simulink model "delayedobserver"  (R2016b)
settings: Solver=ode45  StartTime=0.0  StopTime=T  MaxStep=MaxStep  RelTol=RelTol  EnableMultiTasking=on
values from neighbouring files (symbols this model uses):
  J = 50    [ACC2018_1402_workspace.mat]    (also in initialization.m)
  L = [0.77524 0.18123 -0.12123 -0.17406 0.22469]    [ACC2018_1402_workspace.mat]    (also in initialization.m = [0.77524 0.18123 -0.12123 -0.17406 0.22469]')
  Q = [1 0 0 0 1]    [ACC2018_1402_workspace.mat]    (also in initialization.m)
  rule = 1    [ACC2018_1402_workspace.mat]    (also in initialization.m)
  T = 50    [ACC2018_1402_workspace.mat]    (also in initialization.m)
  T1 = 0.2    [ACC2018_1402_workspace.mat]    (also in initialization.m)
  T2 = 3    [ACC2018_1402_workspace.mat]    (also in initialization.m)
  Tdel = 0.15    [ACC2018_1402_workspace.mat]    (also in initialization.m)
  x0 = [1.73848352419 -6.75635383614 5.88569081368 -3.7756991591 0.570662710124 1 2.03963882803 -4.7405743092 3.08158196954 3.7842900628 4.96303185647 0.0125732066995]    [ACC2018_1402_workspace.mat]    (also in initialization.m = [taus0; e0; mu0; tau0])
libraries: simulink x3
settings Model: Creator=pablonanez  LastModifiedBy=Berk
settings DataIOCC: LimitDataPoints=on  SaveFormat=Array  SignalLoggingSaveFormat=ModelDataLogs
settings OptimizationCC: ExpressionDepthLimit=2147483647  LifeSpan=inf
settings DebuggingCC: UnderspecifiedInitializationDetection=Classic  MergeDetectMultiDrivingBlocksExec=none  SolverPrmCheckMsg=warning  FcnCallInpInsideContextMsg=warning  StateNameClashWarn=warning  SFUnexpectedBacktrackingDiag=warning  SFNoUnconditionalDefaultTransitionDiag=warning  SFExecutionAtInitializationDiag=none
settings HardwareCC: ProdBitPerPointer=32  ProdBitPerSizeT=32  ProdBitPerPtrDiffT=32  ProdLargestAtomicFloat=None  ProdIntDivRoundTo=Undefined  ProdEndianess=Unspecified  ProdWordSize=32  ProdHWDeviceType=32-bit Generic
settings ModelReferenceCC: PropagateSignalLabelsOutOfModel=off
settings SFSimCC: SimParseCustomCode=off
settings GRTTargetCC: TargetLangStandard=C89/C90 (ANSI)  GeneratePreprocessorConditionals=Disable all  CombineOutputUpdateFcns=off  GRTInterface=on
settings ConfigComp: CovMetricSettings=dw  CovHtmlReporting=on  CovSaveCumulativeToWorkspaceVar=on  CovSaveSingleToWorkspaceVar=on  CovExternalEMLEnable=off

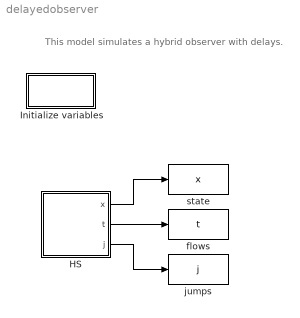
== system delayedobserver ==
  note: This model simulates a hybrid observer with delays.
  HS : Subsystem  LoadFcn=set_param(gcb,'LinkStatus','none')
      settings: CopyFcn=|
      | set_param(gcb,'LinkStatus','none')
      | set_param(gcs, 'MaxStep', 'MaxStep', 'RelTol', 'RelTol')
      mask Display:
      | image(imread('Hcal.jpg'))
      | %plot([5 20 20 5 5],[5 5 20 20 5])
      | %text(8,13,'HyEq_mdl')
      | port_label('output', 1, 'x')
      | port_label('output', 2, 't')
      | port_label('output', 3, 'j')
  Initialize variables : Subsystem  Priority=-10
      settings: OpenFcn=initialization_ex1_4
      mask Display: disp('Double Click\n to Initialize')
  flows : ToWorkspace  VariableName=t  SampleTime=-1
  jumps : ToWorkspace  VariableName=j  SampleTime=-1
  state : ToWorkspace  VariableName=x  SampleTime=-1
  wires:
  HS/1(x) -> state/1
  HS/2(t) -> flows/1
  HS/3(j) -> jumps/1

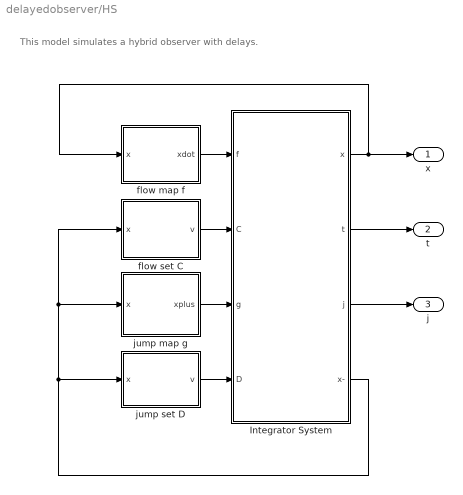
== system delayedobserver/HS ==
  note: This model simulates a hybrid observer with delays.
  Integrator System : Subsystem  Priority=2  mask(Hybrid Integrator){T=T, J=J, x0=x0}
      mask prompts: T "Flow Horizon"; J "Jump Horizon"; x0 "Initial Condition"
      mask help:
      | This block integrates the state of the hybrid system defined by the flow map f (first input), the flow set C (second input), the jump map g (third input) and the jump set D (fourth input).
      | Starting from the initial condition x0 (last mask parameter), the system's state x evolves continuously within the set C, according to f(x,u), but is also subject to jumps within D, according to g(x,u).
      | The block also stops the simulation when the time t is greater than the flow horizon T (first mask parameter), or when the number of jumps j is greater than the jump horizon J (second mask parameter).
      | The outputs of the blocks are respectively x(t), t, j, x(t-).
      mask Help:
      | This block integrates the state of the hybrid system defined by the flow map f (first input), the flow set C (second input), the jump map g (third input) and the jump set D (fourth input).
      | <br>
      | Starting from the initial condition x0 (last mask parameter), the system's state x evolves continuously within the set C, according to f(x,u), but is also subject to jumps within D, according to g(x,u).
      | <br>
      | The block also stops the simulation when the time t is greater than the flow horizon T (first mask parameter), or when the number of jumps j is greater than the jump horizon J (second mask parameter).
      | <br>
      | The outputs of the blocks are respectively x(t), t, j, x(t-).
      | <br>
      | You can right click on the block and "Look under mask" to see what's inside the block.
      | Finally, refer to the manual (HybridSimulator_vXX.pdf) for more detailed information on how this hybrid simulator works.
  flow map f : MATLAB Function  TreatAsAtomicUnit=on
  flow set C : MATLAB Function  TreatAsAtomicUnit=on
  jump map g : MATLAB Function  Priority=2  TreatAsAtomicUnit=on
  jump set D : MATLAB Function  TreatAsAtomicUnit=on
  x : Outport
  t : Outport  Port=2
  j : Outport  Port=3
  wires:
  flow map f/1(xdot) -> Integrator System/1(f)
  Integrator System/4(x-) -> jump set D/1(x), flow set C/1(x), jump map g/1(x)
  Integrator System/1(x) -> flow map f/1(x), x/1
  flow set C/1(v) -> Integrator System/2(C)
  Integrator System/2(t) -> t/1
  Integrator System/3(j) -> j/1
  jump set D/1(v) -> Integrator System/4(D)
  jump map g/1(xplus) -> Integrator System/3(g)

== system delayedobserver/Initialize variables ==

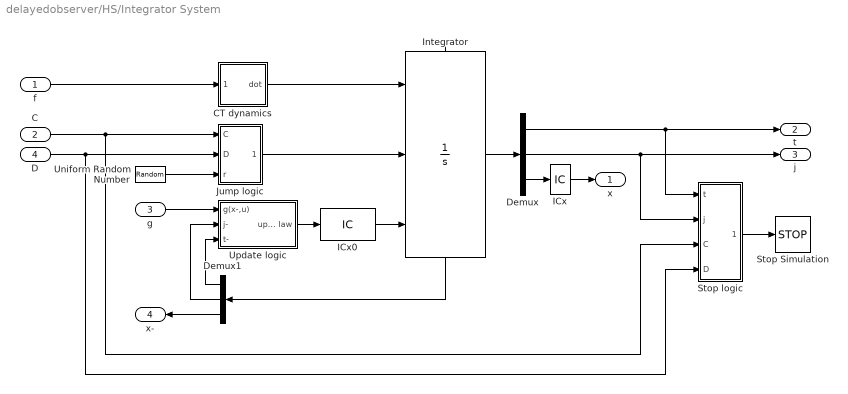
== system delayedobserver/HS/Integrator System ==
  f : Inport
  C : Inport  Port=2
  g : Inport  Port=3
  D : Inport  Port=4
  CT dynamics : Subsystem
  Demux : Demux  Outputs=[1 1 -1]
  Demux1 : Demux  Outputs=[1 1 -1]
  ICx : InitialCondition  Value=x0
  ICx0 : InitialCondition  Value=[0; 0; x0(:)]
  Integrator : Integrator  ExternalReset=level hold  InitialConditionSource=external  ShowStatePort=on  ZeroCross=off
  Jump logic : Subsystem
  Stop Simulation : Stop
  Stop logic : Subsystem
  Uniform Random Number : UniformRandomNumber  Minimum=0  Seed=abs(floor(100*rand))  SampleTime=0
  Update logic : Subsystem
  x : Outport
  t : Outport  Port=2
  j : Outport  Port=3
  x- : Outport  Port=4
  wires:
  Demux1/2 -> Update logic/2(j-)
  Demux1/1 -> Update logic/3(t-)
  g/1 -> Update logic/1(g(x-,u))
  Uniform Random Number/1 -> Jump logic/3(r)
  Jump logic/1(jump) -> Integrator/2
  Demux1/3 -> x-/1
  f/1 -> CT dynamics/1(f(x,u))
  D/1 -> Jump logic/2(D), Stop logic/4(D)
  C/1 -> Jump logic/1(C), Stop logic/3(C)
  Integrator/1 -> Demux/1
  Stop logic/1(stop) -> Stop Simulation/1
  CT dynamics/1(dot) -> Integrator/1
  Update logic/1(update law) -> ICx0/1
  Demux/1 -> Stop logic/1(t), t/1
  Demux/2 -> Stop logic/2(j), j/1
  Integrator/State -> Demux1/1
  Demux/3 -> ICx/1
  ICx/1 -> x/1
  ICx0/1 -> Integrator/3

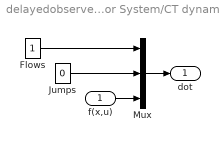
== system delayedobserver/HS/Integrator System/CT dynamics ==
  f(x,u) : Inport
  Flows : Constant
  Jumps : Constant  Value=0
  Mux : Mux  Inputs=[1 1 -1]
  dot : Outport
  wires:
  f(x,u)/1 -> Mux/3
  Mux/1 -> dot/1
  Flows/1 -> Mux/1
  Jumps/1 -> Mux/2

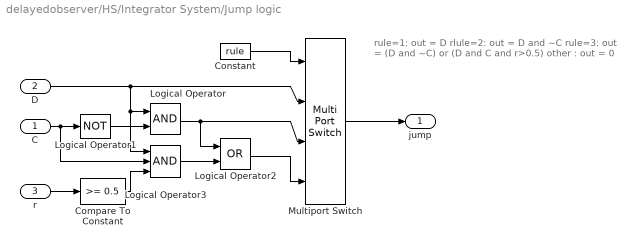
== system delayedobserver/HS/Integrator System/Jump logic ==
  note: rule=1:  out = D
      | rlule=2: out = D and ~C
      | rule=3:  out = (D and ~C)  or (D and C and r>0.5)
      | other :  out = 0
  C : Inport
  D : Inport  Port=2
  r : Inport  Port=3
  Compare To Constant : simulink/Logic and Bit Operations/Compare To Constant  relop=>=  const=0.5  OutDataTypeStr=uint8
  Constant : Constant  Value=rule
  Logical Operator : Logic  AllPortsSameDT=off  OutDataTypeStr=boolean
  Logical Operator1 : Logic  Operator=NOT  Inputs=1  AllPortsSameDT=off  OutDataTypeStr=boolean
  Logical Operator2 : Logic  Operator=OR  AllPortsSameDT=off  OutDataTypeStr=boolean
  Logical Operator3 : Logic  Inputs=3  AllPortsSameDT=off  OutDataTypeStr=boolean
  Multiport Switch : MultiPortSwitch
  jump : Outport
  wires:
  Logical Operator3/1 -> Logical Operator2/2
  Compare To Constant/1 -> Logical Operator3/3
  Multiport Switch/1 -> jump/1
  Logical Operator2/1 -> Multiport Switch/4
  Logical Operator/1 -> Logical Operator2/1, Multiport Switch/3
  Logical Operator1/1 -> Logical Operator/2
  C/1 -> Logical Operator1/1, Logical Operator3/2
  r/1 -> Compare To Constant/1
  D/1 -> Multiport Switch/2, Logical Operator/1, Logical Operator3/1
  Constant/1 -> Multiport Switch/1

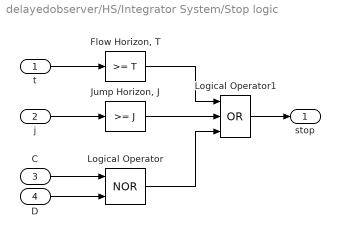
== system delayedobserver/HS/Integrator System/Stop logic ==
  t : Inport
  j : Inport  Port=2
  C : Inport  Port=3
  D : Inport  Port=4
  "Flow Horizon, T" : simulink/Logic and Bit Operations/Compare To Constant  relop=>=  const=T  OutDataTypeStr=uint8  ZeroCross=off
  "Jump Horizon, J" : simulink/Logic and Bit Operations/Compare To Constant  relop=>=  const=J  OutDataTypeStr=uint8  ZeroCross=off
  Logical Operator : Logic  Operator=NOR  AllPortsSameDT=off  OutDataTypeStr=boolean
  Logical Operator1 : Logic  Operator=OR  Inputs=3  AllPortsSameDT=off  OutDataTypeStr=boolean
  stop : Outport
  wires:
  Logical Operator1/1 -> stop/1
  C/1 -> Logical Operator/1
  j/1 -> "Jump Horizon, J"/1
  t/1 -> "Flow Horizon, T"/1
  D/1 -> Logical Operator/2
  Logical Operator/1 -> Logical Operator1/3
  "Jump Horizon, J"/1 -> Logical Operator1/2
  "Flow Horizon, T"/1 -> Logical Operator1/1

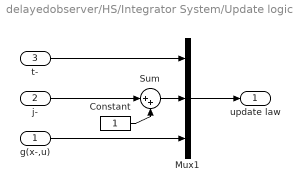
== system delayedobserver/HS/Integrator System/Update logic ==
  g(x-,u) : Inport
  j- : Inport  Port=2
  t- : Inport  Port=3
  Constant : Constant
  Mux1 : Mux  Inputs=[1 1 -1]
  Sum : Sum  Inputs=|++
  update law : Outport
  wires:
  Constant/1 -> Sum/2
  t-/1 -> Mux1/1
  g(x-,u)/1 -> Mux1/3
  j-/1 -> Sum/1
  Mux1/1 -> update law/1
  Sum/1 -> Mux1/2

== matlab function delayedobserver/HS/jump set D ==
  data: x input size=12; v output size=1; eps parameter
function v  = D(x,eps)

%%%%%%%%%%%%%%%%%%%%%%%%%%%%%%%%%%%%%%%%%%%%%%%%%%%%%%%%%%%%%%%%%%%%%%%%%%%
% Matlab Function  Author: Berk Altin
%
% Project: Simulation of a hybrid observer with delays
%
% Name: D.m
%
% Description: Jump set
%
% Version: 1.0
% Required files: -
%%%%%%%%%%%%%%%%%%%%%%%%%%%%%%%%%%%%%%%%%%%%%%%%%%%%%%%%%%%%%%%%%%%%%%%%%%%

% Extract required states
taus = x(1);
tau  = x(12);

% Report jumps if taus \in[-eps,eps]
% or tau \in[-eps,eps]
% eps used instead of 0 for robust simulation
if((abs(taus) <= eps) || (abs(tau) <= eps))
    v = 1;
else
    v = 0;
end
    
end

== matlab function delayedobserver/HS/flow map f ==
  data: x input size=12; xdot output size=12; A parameter
function xdot = f(x,A)

%%%%%%%%%%%%%%%%%%%%%%%%%%%%%%%%%%%%%%%%%%%%%%%%%%%%%%%%%%%%%%%%%%%%%%%%%%%
% Matlab Function  Author: Berk Altin
%
% Project: Simulation of a hybrid observer with delays
%
% Name: f.m
%
% Description: Flow map
%
% Version: 1.0
% Required files: -
%%%%%%%%%%%%%%%%%%%%%%%%%%%%%%%%%%%%%%%%%%%%%%%%%%%%%%%%%%%%%%%%%%%%%%%%%%%

% Extract required states
e    = x(2:6);  % state estimation error
mu   = x(7:11); % memory state
tau  = x(12);   % delay timer

% Assign states
tausdot = -1;
edot = A*e;
mudot = zeros(size(mu));

% Define the flow map f globally--the flow set will be used to restrict it
% for a robust simulation
if (tau >= 0)
    xdot = [tausdot; edot; mudot; -1];
else
    xdot = [tausdot; edot; mudot; 0];
end

end

== matlab function delayedobserver/HS/flow set C ==
  data: x input size=12; v output size=1; Tdel parameter; T2 parameter
function v  = C(x,Tdel, T2)

%%%%%%%%%%%%%%%%%%%%%%%%%%%%%%%%%%%%%%%%%%%%%%%%%%%%%%%%%%%%%%%%%%%%%%%%%%%
% Matlab Function  Author: Berk Altin
%
% Project: Simulation of a hybrid observer with delays
%
% Name: C.m
%
% Description: Flow set
%
% Version: 1.0
% Required files: -
%%%%%%%%%%%%%%%%%%%%%%%%%%%%%%%%%%%%%%%%%%%%%%%%%%%%%%%%%%%%%%%%%%%%%%%%%%%

% Extract required states
taus = x(1);    % sampling timer
tau  = x(12);   % delay timer

% Report flows if taus \in[-eps,T2]
% and tau \in\{0\}\cup[-eps,Tdel]
% -eps used instead of 0 for robust simulation
if((taus >= -eps) && (taus <= T2))
    if(tau==-1)
        v = 1;
    elseif((tau >= -eps) && (tau <= Tdel))
        v = 1;
    else
        v = 0;
    end
else
    v = 0;
end

end

== matlab function delayedobserver/HS/jump map g ==
  data: x input size=12; xplus output size=12; L parameter; Q parameter; T1 parameter; T2 parameter; Tdel parameter
function xplus = g(x,L, Q, T1, T2, Tdel)

%%%%%%%%%%%%%%%%%%%%%%%%%%%%%%%%%%%%%%%%%%%%%%%%%%%%%%%%%%%%%%%%%%%%%%%%%%%
% Matlab Function  Author: Berk Altin
%
% Project: Simulation of a hybrid observer with delays
%
% Name: g.m
%
% Description: Jump map
%
% Version: 1.0
% Required files: -
%%%%%%%%%%%%%%%%%%%%%%%%%%%%%%%%%%%%%%%%%%%%%%%%%%%%%%%%%%%%%%%%%%%%%%%%%%%

% Extract required states
taus = x(1);    % sampling timer
e    = x(2:6);  % state estimation error
mu   = x(7:11); % memory state
tau  = x(12);   % delay timer

% Randomly select the arrival of the next sample
r           = rand(1);
tausplus    = r*T1+(1-r)*T2;

eplus       = (eye(5)-L*Q)*e;
xplus = x;

% define the jump map g "globally"--the jump set will be used to restrict
% it for a robust simulation
% bounds on tau (-0.75) and taus (-0.5) again for robustness
if (tau <= -0.75)       % if tau = -1, consider g for the case taus = 0
    xplus = [tausplus; e; eplus; Tdel];
elseif (tau >= -0.5)    % if tau = 0, no jumps due to taus = 0
    xplus = [taus; mu; mu; -1];
end

end
